simulink model "drone_model"  (R2019a)
settings: Solver=VariableStepAuto  StartTime=0.0  StopTime=10.0  RelTol=1e-3
values from neighbouring files (symbols this model uses):
  drag_coefficient = 0    [drone_simulation.m]
  input1 = 1    [drone_simulation.m]
  input2 = 2    [drone_simulation.m]
  input3 = 3    [drone_simulation.m]
  input4 = 4    [drone_simulation.m]
  thrust_coefficient = 200    [drone_simulation.m]
libraries: dspinverses x1
settings Model: Creator=Jeff  LastModifiedBy=Jeff

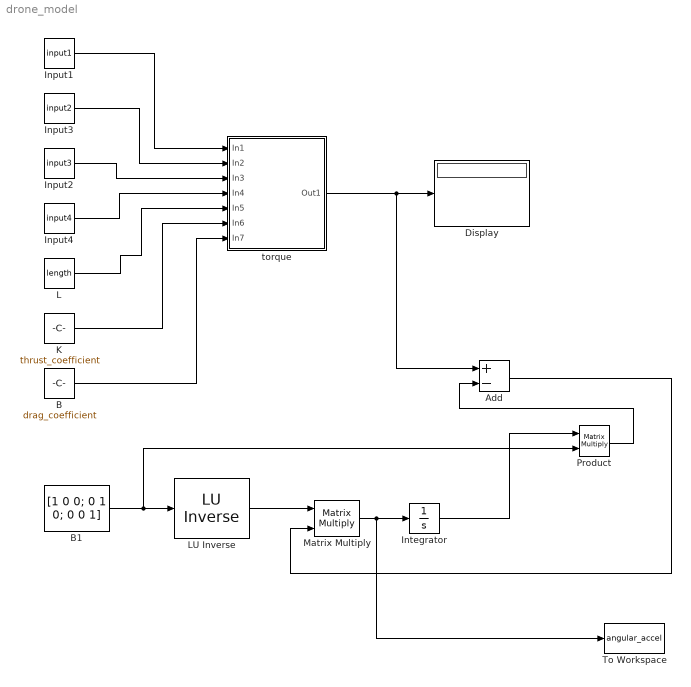
== system drone_model ==
  " LU Inverse" : dspinverses/ LU Inverse
      settings: SourceProductName=DSP System Toolbox
  Add : Sum  Inputs=+-
  B : Constant  Value=drag_coefficient
  B1 : Constant  Value=[1 0 0; 0 1 0; 0 0 1]
  Display : Display
  Input1 : Constant  Value=input1
  Input2 : Constant  Value=input3
  Input3 : Constant  Value=input2
  Input4 : Constant  Value=input4
  Integrator : Integrator
  K : Constant  Value=thrust_coefficient
  L : Constant  Value=length
  Matrix Multiply : Product  Multiplication=Matrix(*)
  Product : Product  Multiplication=Matrix(*)
  To Workspace : ToWorkspace  VariableName=angular_accel  SampleTime=-1
  torque : Subsystem
  wires:
  Input1/1 -> torque/1(In1)
  Input3/1 -> torque/2(In2)
  Input2/1 -> torque/3(In3)
  Input4/1 -> torque/4(In4)
  L/1 -> torque/5(In5)
  K/1 -> torque/6(In6)
  B/1 -> torque/7(In7)
  torque/1(Out1) -> Add/1, Display/1
  B1/1 -> Product/2, " LU Inverse"/1
  " LU Inverse"/1 -> Matrix Multiply/1
  Matrix Multiply/1 -> To Workspace/1, Integrator/1
  Integrator/1 -> Product/1
  Product/1 -> Add/2
  Add/1 -> Matrix Multiply/2

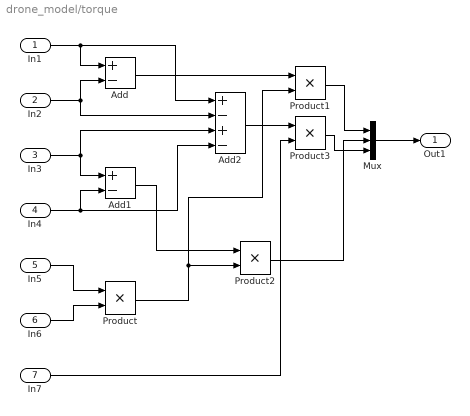
== system drone_model/torque ==
  In1 : Inport
  In2 : Inport  Port=2
  In3 : Inport  Port=3
  In4 : Inport  Port=4
  In5 : Inport  Port=5
  In6 : Inport  Port=6
  In7 : Inport  Port=7
  Add : Sum  Inputs=+-
  Add1 : Sum  Inputs=+-
  Add2 : Sum  Inputs=+-+-
  Mux : Mux  Inputs=3
  Product{,1..3} (4 alike) : Product
  Out1 : Outport
  wires:
  In1/1 -> Add2/1, Add/1
  In4/1 -> Add1/2, Add2/4
  In5/1 -> Product/1
  In2/1 -> Add2/2, Add/2
  Add1/1 -> Product2/1
  Mux/1 -> Out1/1
  Add/1 -> Product1/1
  Product/1 -> Product1/2, Product2/2
  In3/1 -> Add1/1, Add2/3
  In6/1 -> Product/2
  Product3/1 -> Mux/3
  Product2/1 -> Mux/2
  Product1/1 -> Mux/1
  Add2/1 -> Product3/1
  In7/1 -> Product3/2
